simulink model "projectp4"  (R2020a)
settings: Solver=VariableStepAuto  StartTime=0.0  StopTime=10.0  RelTol=1e-3
undefined symbols (not defined in the file or in its folder): i_ss, m, y_ss
settings Model: Creator=Joey Baby  LastModifiedBy=Joey Baby

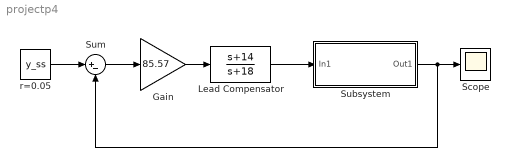
== system projectp4 ==
  Gain : Gain  Gain=85.57
  Lead Compensator : TransferFcn  Numerator=[1 14]  Denominator=[1 18]
  Scope : Scope
  Subsystem : Subsystem
  Sum : Sum  Inputs=|+-
  r=0.05 : Constant  Value=y_ss
  wires:
  r=0.05/1 -> Sum/1
  Sum/1 -> Gain/1
  Gain/1 -> Lead Compensator/1
  Subsystem/1(Out1) -> Sum/2, Scope/1
  Lead Compensator/1 -> Subsystem/1(In1)

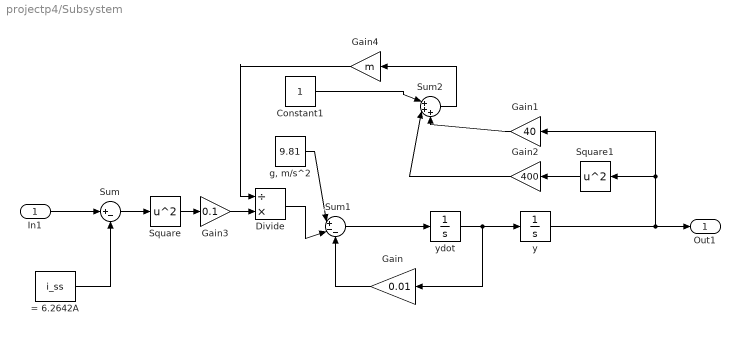
== system projectp4/Subsystem ==
  In1 : Inport
  = 6.2642A : Constant  Value=i_ss
  Constant1 : Constant
  Divide : Product  Inputs=/*
  Gain : Gain  Gain=0.01
  Gain1 : Gain  Gain=40
  Gain2 : Gain  Gain=400
  Gain3 : Gain  Gain=0.1
  Gain4 : Gain  Gain=m
  Square : Math  Operator=square  SaturateOnIntegerOverflow=on
  Square1 : Math  Operator=square  SaturateOnIntegerOverflow=on
  Sum : Sum  Inputs=|+-
  Sum1 : Sum  Inputs=|+--
  Sum2 : Sum  Inputs=|+++
  "g, m/s^2" : Constant  Value=9.81
  y : Integrator  InitialCondition=1.7
  ydot : Integrator  InitialCondition=0.1
  Out1 : Outport
  wires:
  In1/1 -> Sum/1
  = 6.2642A/1 -> Sum/2
  Sum/1 -> Square/1
  Square/1 -> Gain3/1
  Divide/1 -> Sum1/2
  Sum2/1 -> Gain4/1
  ydot/1 -> Gain/1, y/1
  Gain/1 -> Sum1/3
  Constant1/1 -> Sum2/1
  y/1 -> Square1/1, Gain1/1, Out1/1
  "g, m/s^2"/1 -> Sum1/1
  Gain2/1 -> Sum2/2
  Gain1/1 -> Sum2/3
  Square1/1 -> Gain2/1
  Sum1/1 -> ydot/1
  Gain3/1 -> Divide/2
  Gain4/1 -> Divide/1
